simulink model "TRN_V3_2"  (R2022a)
settings: Solver=FixedStepAuto  StartTime=0.0  StopTime=300  FixedStep=0.04  RelTol=1e-3
PreLoadFcn:
  | load('BusStructureTRNsensor.mat');
  | addpath('C:/MAP');
InitFcn:
  | %load TRNDataBusPILS.mat
  | %addpath(genpath(cd))
  | 
  | %load('TPF_WHOLESIM_INPUT_SCENARIOS_AGCAS_N35_10E127_70.mat');
  | 
  | % Add DataBus Path
  | addpath(',,/');
  | addpath('../MAP/');
  | addpath('../MAP/MAP_DB');
  | addpath('../MAP/DVOF');
  | addpath(genpath(cd));
  | load('BusStructureTRN.mat');
undefined symbols (not defined in the file or in its folder): Altitude_INS, Latitude_INS, Longitude_INS, residual, Result_Prev, TimeTag_Prev, TRN, TRNlib
libraries: simulink_extras x21, sharedtransform x2
(part 3 of 4)

== system TRN_V3_2/TRN/ModeManagementCSU/TrackingCSU/TrackingCSU_20230430/TrackingCSU_Measurement/Measurement_GPSinvalid/residualValidCheck ==
  TRNDatapump : Inport
  Bus Selector7 : BusSelector  OutputSignals=residual
  Data Type Conversion2 : DataTypeConversion  OutDataTypeStr=boolean  SaturateOnIntegerOverflow=off  RndMeth=Floor
  Demux : Demux  Outputs=2
  Gain2 : Gain  Gain=3
  StdDev : MATLAB Function  TreatAsAtomicUnit=on
  Terminator : Terminator
  Unit Delay3 : UnitDelay  SampleTime=-1  HasFrameUpgradeWarning=on
  residualCheck : MATLAB Function  TreatAsAtomicUnit=on
  residualValid : Outport
  wires:
  Data Type Conversion2/1 -> residualValid/1
  residualCheck/1(residualValid) -> Data Type Conversion2/1
  StdDev/1(std) -> Gain2/1
  Gain2/1 -> residualCheck/2(sigma_3)
  residualCheck/2(count) -> Unit Delay3/1
  TRNDatapump/1 -> Bus Selector7/1
  Unit Delay3/1 -> residualCheck/3("count ")
  Bus Selector7/1 -> Demux/1  "<residual>"
  Demux/1 -> residualCheck/1(residual), StdDev/1(x)
  Demux/2 -> Terminator/1

== system TRN_V3_2/TRN/ModeManagementCSU/TrackingCSU/TrackingCSU_20230430/TrackingCSU_Measurement/Measurement_GPSvalid/residualValidCheck ==
  TRNDatapump : Inport
  Bus Selector7 : BusSelector  OutputSignals=residual
  Data Type Conversion2 : DataTypeConversion  OutDataTypeStr=boolean  SaturateOnIntegerOverflow=off  RndMeth=Floor
  Demux : Demux  Outputs=2
  Gain2 : Gain  Gain=3
  StdDev : MATLAB Function  TreatAsAtomicUnit=on
  Terminator : Terminator
  Unit Delay3 : UnitDelay  SampleTime=-1  HasFrameUpgradeWarning=on
  residualCheck : MATLAB Function  TreatAsAtomicUnit=on
  residualValid : Outport
  wires:
  Unit Delay3/1 -> residualCheck/3("count ")
  TRNDatapump/1 -> Bus Selector7/1
  residualCheck/2(count) -> Unit Delay3/1
  Gain2/1 -> residualCheck/2(sigma_3)
  StdDev/1(std) -> Gain2/1
  residualCheck/1(residualValid) -> Data Type Conversion2/1
  Data Type Conversion2/1 -> residualValid/1
  Bus Selector7/1 -> Demux/1  "<residual>"
  Demux/2 -> residualCheck/1(residual), StdDev/1(x)
  Demux/1 -> Terminator/1

== matlab function TRN_V3_2/TRN/ModeManagementCSU/TrackingCSU/TrackingCSU_20230430/TrackingCSU_ConvertInput1/GPSflagcheck ==
  data: FoM input; GPSflag output; GPSDataNotValid input; AccY input
function GPSflag  = GPScheck(FoM, GPSDataNotValid, AccY)

GPSflag = uint32(2);

if GPSDataNotValid == 0
%     if EstHorErr < 100 && EstVerErr < 25 && state == 5
        if FoM <= 4
            GPSflag = uint32(1);
            if FoM <= 2 && abs(AccY) < 2
                GPSflag = uint32(0);
            end
        end
%    end
else
    GPSflag = uint32(2);
end

== matlab function TRN_V3_2/TRN/ModeManagementCSU/TrackingCSU/TrackingCSU_20230430/TrackingCSU_Measurement/Measurement_GPSinvalid/MATLAB Function ==
  data: Rmat output
function Rmat = Rmatrix_GPSinvalid

% Original
% Rmat = diag((35/sqrt(25))^2);

% Monte-carlo simulation 972
% use min data
Rmat = diag((12.0679/sqrt(25))^2);

% Monte-carlo simulation 972
% use mean data
% Rmat = diag((9.9924/sqrt(25))^2);

== matlab function TRN_V3_2/TRN/ModeManagementCSU/TrackingCSU/TrackingCSU_20230430/TrackingCSU_EKFupdate1/EKFUpdate_GPSinvalid/EKFUpdate_GPSinvalid1 ==
  data: zmat_TRN input; xu output; P output; Fmatrix input; Hmat_TRN input; Gmatrix input; P input; Q input; Rmat_TRN input; dt input; residual output; latINSErrTRN output; lonINSErrTRN output; altINSErrTRN output; xu_prev input; TimeTag_Prev input; hUncertainty output; vUncertainty output
function [xu, P, residual, latINSErrTRN, lonINSErrTRN, altINSErrTRN, hUncertainty, vUncertainty] ...
    = EKFUpdate_GPSinvalid(zmat_TRN, Fmatrix, Hmat_TRN, Gmatrix, P, Q, Rmat_TRN, dt, xu_prev, TimeTag_Prev)

x = zeros(15,1);
I = eye(max(size(Fmatrix)));

A = I + (Fmatrix*dt);
Q = (A*Gmatrix * Q * Gmatrix'*A') .* dt;

%-------------------------------------%
% Predicts states & covariance matrix
%-------------------------------------%
xp = A * x;
Pp = (A * P * A') + Q;


K = (Pp * Hmat_TRN')/(Rmat_TRN + Hmat_TRN * Pp * Hmat_TRN');
xu = xp + K * (zmat_TRN - Hmat_TRN*xp);
residual = zmat_TRN;
P = (I - K*Hmat_TRN) * Pp * (I - K*Hmat_TRN)' + K*Rmat_TRN*K';

hUncertainty = sqrt(abs(P(7,7) + P(8,8))) * 6378000;    % unit m
vUncertainty = sqrt(abs(P(9,9)));                       % unit m

%---------------------------%
% Updates covariance matrix
%---------------------------%
% P = (I - K*H) * Pp * (I - K*H)' + K*R*K';

latINSErrTRN = xu(7);
lonINSErrTRN = xu(8);
altINSErrTRN = xu(9);

if (TimeTag_Prev(6) == 1)
    xu = xu_prev;
    latINSErrTRN = xu(7);
    lonINSErrTRN = xu(8);
    altINSErrTRN = xu(9);
end

== matlab function TRN_V3_2/TRN/ModeManagementCSU/TrackingCSU/TrackingCSU_20230430/TrackingCSU_Measurement/Measurement_GPSvalid/Rmat_GPS_v1 ==
  data: FoM input; Rmat output
% Original

function Rmat = Rmat_GPS(FoM)
Pcode = false;
if Pcode == true
    a = 6.4029;
    b = 6.7450;
    c = 8.8381;
    d = 0.8866;
    e = 1.1000;
    f = 3.3142;
elseif FoM == 1
    a = 6.4266;
    b = 6.7548;
    c = 17.6319;
    d = 0.8866;
    e = 1.1000;
    f = 3.3142;
elseif FoM == 2
    a = 6.5362;
    b = 6.8383;
    c = 34.2994;
    d = 0.8866;
    e = 1.1000;
    f = 3.3142;
elseif FoM == 3
    a = 6.7864;
    b = 7.0654;
    c = 55.6432;
    d = 0.8866;
    e = 1.1000;
    f = 3.3142;
elseif FoM == 4
    a = 7.1520;
    b = 7.4164;
    c = 77.1714;
    d = 0.8866;
    e = 1.1000;
    f = 3.3142;
else
    a = 8.6486;
    b = 8.8154;
    c = 135.9654;
    d = 0.8866;
    e = 1.1000;
    f = 3.3142;
end

Rmat = diag([ (a/sqrt(25))^2 (b/sqrt(25))^2 (c/sqrt(25))^2 (d/sqrt(25))^2 (e/sqrt(25))^2 (f/sqrt(25))^2 ]);

% Rmat = diag([ (6.6/sqrt(25))^2 (6.6/sqrt(25))^2 (1/sqrt(25))^2 (0.5/sqrt(25))^2 (0.5/sqrt(25))^2 (0.5/sqrt(25))^2 ]);

== matlab function TRN_V3_2/TRN/ModeManagementCSU/TrackingCSU/TrackingCSU_20230430/TrackingCSU_EKFupdate1/EKFUpdate_GPSinvalid/EKFUpdate_Predict_GPSinvalid ==
  data: I output; Zmat_GPSinvalid input; xp output; Pp output; Fmatrix input; Hmat_GPSinvalid input; Gmatrix input; P input; Q input; Rmat_GPSinvalid input; dt input; residual_GPSinvalid output; K output
function [I, xp, Pp, residual_GPSinvalid, K] ...
    = EKFUpdate_Predict_GPSinvalid(Zmat_GPSinvalid, Fmatrix, Hmat_GPSinvalid, Gmatrix, P, Q, Rmat_GPSinvalid, dt)

x = zeros(15,1);
I = eye(max(size(Fmatrix)));

A = I + (Fmatrix*dt);
Q = (A*Gmatrix * Q * Gmatrix'*A') .* dt;

%-------------------------------------%
% Predicts states & covariance matrix
%-------------------------------------%
xp = A * x;
Pp = (A * P * A') + Q;


K = (Pp * Hmat_GPSinvalid')/(Rmat_GPSinvalid + Hmat_GPSinvalid * Pp * Hmat_GPSinvalid');
residual_GPSinvalid = Zmat_GPSinvalid;

== matlab function TRN_V3_2/TRN/ModeManagementCSU/TrackingCSU/TrackingCSU_20230430/TrackingCSU_Measurement/Measurement_GPSvalid/Rmat_GPS_v2 ==
  data: FoM input; Rmat output
% Monte-carlo simulation 972
% use mean data

function Rmat = Rmat_GPS(FoM)
Pcode = false;
if Pcode == true
    a = 45.9175;
    b = 46.6241;
    c = 10.2589;
    d = 0.1085;
    e = 0.1108;
    f = 0.5579;
elseif FoM == 1
    a = 46.7399;
    b = 47.4166;
    c = 18.7833;
    d = 0.1085;
    e = 0.1108;
    f = 0.5579;
elseif FoM == 2
    a = 49.2325;
    b = 49.8506;
    c = 35.6076;
    d = 0.1085;
    e = 0.1108;
    f = 0.5579;
elseif FoM == 3
    a = 53.5206;
    b = 54.0688;
    c = 56.2876;
    d = 0.1085;
    e = 0.1108;
    f = 0.5579;
elseif FoM == 4
    a = 58.8912;
    b = 59.3679;
    c = 77.2285;
    d = 0.1085;
    e = 0.1108;
    f = 0.5579;
else
    a = 58.8912;
    b = 59.3679;
    c = 77.2285;
    d = 0.1085;
    e = 0.1108;
    f = 0.5579;
end

Rmat = diag([ (a/sqrt(25))^2 (b/sqrt(25))^2 (c/sqrt(25))^2 (d/sqrt(25))^2 (e/sqrt(25))^2 (f/sqrt(25))^2 ]);

== matlab function TRN_V3_2/TRN/ModeManagementCSU/ValidityCheck/ValidityCheck ==
  data: continuousValid input; TRNEstOfINSLatitudeErr output; TRNEstOfINSLongitudeErr output; TRNEstOfINSAltitudeErr output; AircraftPositionCorrectionValid output; latINSErrTRN input; lonINSErrTRN input; altINSErrTRN input; velFlag input
function [TRNEstOfINSLatitudeErr, TRNEstOfINSLongitudeErr, TRNEstOfINSAltitudeErr, AircraftPositionCorrectionValid] = ...
    ValidityCheck(continuousValid, latINSErrTRN, lonINSErrTRN, altINSErrTRN, velFlag)

if continuousValid == true || velFlag == true
    TRNEstOfINSLatitudeErr = latINSErrTRN * 180/pi;
    TRNEstOfINSLongitudeErr = lonINSErrTRN * 180/pi;
    TRNEstOfINSAltitudeErr = altINSErrTRN;
    AircraftPositionCorrectionValid = true;
else
    TRNEstOfINSLatitudeErr = 0.0;
    TRNEstOfINSLongitudeErr = 0.0;
    TRNEstOfINSAltitudeErr = 0.0;
    AircraftPositionCorrectionValid = false;
end
end

== matlab function TRN_V3_2/TRN/ModeManagementCSU/TrackingCSU/TrackingCSU_20230430/TrackingCSU_Measurement/Fupdate ==
  data: velN input; Fmatrix output; velE input; velD input; lat input; alt input; accN input; accE input; accD input; OM input; M input; N input; DCMbn input
% ---------------------------------------------------------------------- %
%                   F matrix update function
%
%   INPUT:
%       velN: North Velocity                                [m/s]
%       velE: East Velocity                                 [m/s]
%       velD: Down Velocity                                 [m/s]
%       lat: Latitude                                       [rad]
%       alt: Altitude                                       [m]
%       accN: North acceleration                            [m/ss]
%       accE: East acceleration                             [m/ss]
%       accD: Down acceleration                             [m/ss]
%       OM: Magnitude of the rotation rate of the Earth     [rad/s]
%       R0: Radius of Earth                                 [m]
%       DCMbn: Rotational matrix(body frame to navigation frame)
%
%   OUTPUT:
%       Fmatrix: System matrix of Kalman Filter
%
% ---------------------------------------------------------------------- %
function Fmatrix = Fupdate(velN, velE, velD, lat, alt, accN, accE, accD, OM, M, N, DCMbn)
    
        Z  = zeros(3);
    
        e11 = 0;
        e12 = -((OM * sin(lat)) + (velE/(N+alt) * tan(lat)));
        e13 = velN/(M+alt);
        e21 = ((OM * sin(lat)) + (velE/(N+alt) * tan(lat)));
        e22 = 0;
        e23 = ((OM * cos(lat)) + (velE/(N+alt)));
        e31 = -velN/(M+alt);
        e32 = -(OM * cos(lat)) - (velE/(N+alt));
        e33 = 0;
        Fee = [e11 e12 e13; e21 e22 e23; e31 e32 e33;];
    
        e11 = 0;
        e12 = 1/((N+alt));
        e13 = 0;
        e21 = -1/((M+alt));
        e22 = 0 ;
        e23 = 0 ;
        e31 = 0 ;
        e32 = -tan(lat)/(N+alt) ;
        e33 = 0 ;
        Fev = [e11 e12 e13; e21 e22 e23; e31 e32 e33;];
    
        e11 = -OM * sin(lat);
        e12 = 0;
        e13 = -velE/(((N+alt))^2);
        e21 = 0 ;
        e22 = 0 ;
        e23 = velN/(((M+alt))^2);
        e31 =  -(OM*cos(lat)) - (velE/(((N+alt))*(cos(lat))^2));
        e32 = 0 ;
        e33 = (velE * tan(lat)) / ((N+alt)^2) ;
        Fep = [e11 e12 e13; e21 e22 e23; e31 e32 e33;];
    
        e11 = 0 ;
        e12 = -accD ;
        e13 = accE ;
        e21 = accD ;
        e22 = 0 ;
        e23 = -accN ;
        e31 = -accE ;
        e32 = accN ;
        e33 = 0 ;
        Fve = [e11 e12 e13; e21 e22 e23; e31 e32 e33;];
    
        e11 = velD/((M+alt));
        e12 = -2*((OM * sin(lat)) + ((velE/((N+alt))) * tan (lat))) ;
        e13 = velN/(M+alt) ;
        e21 = (2*OM * sin(lat)) + ( (velE/((N+alt))) * tan(lat) );
        e22 = (1/((N+alt))) * ((velN * tan(lat)) + velD) ;
        e23 = 2*OM * cos(lat) + (velE/((N+alt)));
        e31 = (-2*velN)/((M+alt));
        e32 = -2*(OM * cos(lat) +  (velE/((N+alt)))) ;
        e33 = 0;
        Fvv = [e11 e12 e13; e21 e22 e23; e31 e32 e33;];
    
        e11 = -velE*( (2*OM * cos(lat)) + (velE/(((N+alt))*(cos(lat))^2)));
        e12 = 0 ;
        e13 = (((velE^2)*tan(lat))/((N+alt)^2)) - ((velN*velD)/((M+alt)^2)) ;
        e21 = 2*OM *((velN*cos(lat)) - (velD*sin(lat))) + ((velN*velE) / (((N+alt))*(cos(lat))^2)) ;
        e22 = 0 ;
        e23 = ((-velE*velD)/((N+alt)^2))-((velN*velE*tan(lat))/((N+alt)^2));
        e31 = 2 * OM * velE * sin(lat);
        e32 = 0;
        e33 =  (((velE^2)/((N+alt)^2)) + ((velN^2)/((M+alt)^2)));
        Fvp = [e11 e12 e13; e21 e22 e23; e31 e32 e33;];
    
        Fpe = zeros(3);
    
        e11 = 1/((M+alt));
        e12 = 0;
        e13 = 0;
        e21 = 0;
        e22 = 1/(((N+alt))*cos(lat));
        e23 = 0;
        e31 = 0;
        e32 = 0;
        e33 = -1;
        Fpv = [e11 e12 e13; e21 e22 e23; e31 e32 e33;];
    
        e11 = 0;
        e12 = 0;
        e13 = -velN/(((M+alt))^2);
        e21 = (velE*tan(lat))/(((N+alt))*cos(lat));
        e22 = 0;
        e23 = -velE/((((N+alt))^2)*cos(lat));
        e31 = 0;
        e32 = 0;
        e33 = 0;
        Fpp = [e11 e12 e13; e21 e22 e23; e31 e32 e33;];
    
    
        %     Fvv = zeros(3);
        %     Fvp = zeros(3);
        %     Fpp = zeros(3);
    
        Fmatrix =  [Fee    Fev    Fep      DCMbn          Z      ;
                    Fve    Fvv    Fvp        Z           DCMbn   ;
                    Fpe    Fpv    Fpp        Z            Z      ;
                    Z      Z      Z          Z            Z      ;
                    Z      Z      Z          Z            Z      ;];


end

== matlab function TRN_V3_2/TRN/ModeManagementCSU/TrackingCSU/TrackingCSU_20230430/TrackingCSU_Measurement/Gupdate ==
  data: DCMbn input; Gmatrix output
% ---------------------------------------------------------------------- %
%                   G matrix update function
%
%   INPUT:
%       DCMbn: Rotational matrix(body frame to navigation frame)
%
%   OUTPUT:
%       Gmatrix: Input matrix of Kalman Filter
%
% ---------------------------------------------------------------------- %
function Gmatrix = Gupdate(DCMbn)

Z  = zeros(3);

Gmatrix =  [ -DCMbn     Z;
                Z      DCMbn;
                Z       Z;
                Z       Z;
                Z       Z;];      

end

== matlab function TRN_V3_2/TRN/ModeManagementCSU/TrackingCSU/TrackingCSU_20230430/TrackingCSU_Measurement/Measurement_GPSinvalid/MesurementUpdate_GPSinvalid ==
  data: Hmat_GPSinvalid output; lat input; lon input; alt input; RALTAltitude input; Zmat_GPSinvalid output; resolution input
% function [Hmatrix, z, hDEM] = MeasurementUpdate(resolution, lat, lon, alt, RALT)
function [Hmat_GPSinvalid, Zmat_GPSinvalid] = MeasurementUpdate(lat, lon, alt, RALTAltitude, resolution)
    P_low = 0.0;
    P_high = 0.0;    
    P_left = 0.0;    
    P_right = 0.0;
    hDEM = double(0.0);         
    resultDTED = uint32(1);

    lat = rad2deg(lat);
    lon = rad2deg(lon);

    resultDTED = coder.ceval('UpdateCache', lat, lon);
    
    P_low    =   coder.ceval('MAPGetTerrainHeight', lat - resolution, lon);
    P_high   =   coder.ceval('MAPGetTerrainHeight', lat + resolution, lon);
    P_left   =   coder.ceval('MAPGetTerrainHeight', lat, lon - resolution);
    P_right  =   coder.ceval('MAPGetTerrainHeight', lat, lon + resolution);
    
    hdot_lat    =   (P_high - P_low) / (resolution);
    hdot_lon    =   (P_right - P_left) / (resolution);
    
    % H matrix
    Hmat_GPSinvalid = [ zeros(1,6) -hdot_lat   -hdot_lon    1  zeros(1,6) ]; 
    
    hDEM = coder.ceval('MAPGetTerrainHeight', lat, lon);
    
    Zmat_GPSinvalid = (alt - hDEM) - RALTAltitude;

end

== matlab function TRN_V3_2/TRN/ModeManagementCSU/TrackingCSU/TrackingCSU_20230430/TrackingCSU_Measurement/Measurement_GPSinvalid/MesurementValid_GPSinvalid ==
  data: updateValid input; roll input; pitch input; zmat_out output; zmat_in input; RALTTimeTag input; RALTTimeTag_temp input; RLATvalid input
function zmat_out  = MesurementValid(updateValid, roll, pitch, zmat_in, RALTTimeTag, RALTTimeTag_temp, RLATvalid)

zmat_out = 0;

if (updateValid == true && abs(roll) < deg2rad(15) && abs(pitch) < deg2rad(15) && RLATvalid == true && (abs(RALTTimeTag - RALTTimeTag_temp)) ~= 0)
% if (residualValid == true && abs(roll) < deg2rad(15) && abs(pitch) < deg2rad(15) && (abs(RALTTimeTag - RALTTimeTag_temp)) > 0.000000001)
% if (RALTValid == true && abs(roll) < deg2rad(15) && abs(pitch) < deg2rad(15))
    zmat_out = zmat_in;


else
    zmat_out = 0;

end

end

== matlab function TRN_V3_2/TRN/ModeManagementCSU/TrackingCSU/TrackingCSU_20230430/TrackingCSU_Measurement/Measurement_GPSinvalid/residualValidCheck/StdDev ==
  data: x input; std output
function std = StdDev(x)

persistent sumX sumX2 cnt
if (isempty(sumX))
    sumX = 0;
end
if (isempty(sumX2))
    sumX2 = 0;
end
if (isempty(cnt))
    cnt = 0;
end

cnt = cnt + 1;
sumX = sumX + x;
sumX2 = sumX2 + x^2;

var = sumX2/cnt - (sumX/cnt)^2;
std = sqrt(abs(var));
end

== matlab function TRN_V3_2/TRN/ModeManagementCSU/TrackingCSU/TrackingCSU_20230430/TrackingCSU_Measurement/Measurement_GPSinvalid/residualValidCheck/residualCheck ==
  data: residual input; sigma_3 input; residualValid output; count output; count input
function [residualValid, count] = residualCheck(residual, sigma_3, count)

if abs(residual) > sigma_3
    count = count + 1;
else
    count = 0;
end

if count > 7
    residualValid = boolean(false);
else
    residualValid = boolean(true);
end

== matlab function TRN_V3_2/TRN/ModeManagementCSU/TrackingCSU/TrackingCSU_20230430/TrackingCSU_Measurement/Measurement_GPSvalid/Earth_radius ==
  data: M output; N output; psi output; Latitude_INS input
function [M, N, psi] = Earth_radius(Latitude_INS)

    a   = 6378137;          % Earth's equatorial radius
    b   = 6356752.314245;   % Earth's polar radius
    psi = Latitude_INS;     % psi(latitude_INS)
    M   = ((a*b)^2) / ( ( (a*cos(psi))^2 + (b*sin(psi))^2 )^(3/2) );    % radius  of  curvature  in  meridian
    N   = (a^2) / ( ( (a*cos(psi))^2 + (b*sin(psi))^2 )^(1/2) );        % radius  of  curvature  in  prime  vertical

end

== matlab function TRN_V3_2/TRN/ModeManagementCSU/TrackingCSU/TrackingCSU_20230430/TrackingCSU_Measurement/Measurement_GPSvalid/MesurementUpdate_GPSvalid ==
  data: Lat_GPS input; Hmat_GPSvalid output; Lon_GPS input; z_GPSvalid output; Alt_GPS input; velN_GPS input; velE_GPS input; velD_GPS input; Lat_INS input; Lon_INS input; Alt_INS input; velN_INS input; velE_INS input; velD_INS input; M input; N input; psi input
function [Hmat_GPSvalid, z_GPSvalid] = MeasurementUpdate(Lat_GPS, Lon_GPS, Alt_GPS, velN_GPS, velE_GPS, velD_GPS, ...
                                          Lat_INS, Lon_INS, Alt_INS, velN_INS, velE_INS, velD_INS, ...
                                          M, N, psi)
    Z   = zeros(3);
    I   = eye(3);
    H   = [(M+Alt_INS)        0             0;
        0     (N+Alt_INS)*cos(psi)     0;
        0            0             1];

    % H matrix
    Hmat_GPSvalid = [Z Z H Z Z
                   Z I Z Z Z];


    z_GPSvalid = [(M+Alt_INS)*(Lat_INS-Lat_GPS);
        (N+Alt_INS)*cos(psi)*(Lon_INS-Lon_GPS);
        Alt_INS - Alt_GPS;
        velN_INS - velN_GPS;
        velE_INS - velE_GPS;
        velD_INS - velD_GPS];

end

== matlab function TRN_V3_2/TRN/ModeManagementCSU/TrackingCSU/TrackingCSU_20230430/TrackingCSU_Measurement/Measurement_GPSvalid/MesurementValid_GPSvalid ==
  data: zmat_in_GPSvalid input; roll input; pitch input; zmat_GPSvalid output; GPStimeValid input; GPStimeValid_temp input; GPS_flag input; residualValid input
function zmat_GPSvalid = MesurementValid(zmat_in_GPSvalid,  roll, pitch, GPStimeValid, GPStimeValid_temp, GPS_flag, residualValid)

zmat_GPSvalid = zeros(6,1);

if (residualValid == true && abs(roll) < deg2rad(15) && abs(pitch) < deg2rad(15) && (abs(GPStimeValid - GPStimeValid_temp)) ~= 0)
    %     if (residualValid == true) && (abs(GPStimeValid - GPStimeValid_temp) > 0.000000001)

    if GPS_flag == 0
        zmat_GPSvalid = zmat_in_GPSvalid;

    elseif GPS_flag == 1

        for i = 1:6
            zmat_GPSvalid(i) = zmat_in_GPSvalid(i);

            if i > 3
                zmat_GPSvalid(i) = 0;
            end
        end

    else
        zmat_GPSvalid = zeros(6,1);
    end

else
    zmat_GPSvalid = zeros(6,1);

end

end

== matlab function TRN_V3_2/TRN/ModeManagementCSU/TrackingCSU/TrackingCSU_20230430/TrackingCSU_Measurement/Measurement_GPSvalid/residualValidCheck/StdDev ==
  data: x input; std output
function std = StdDev(x)

persistent sumX sumX2 cnt
if (isempty(sumX))
    sumX = 0;
end
if (isempty(sumX2))
    sumX2 = 0;
end
if (isempty(cnt))
    cnt = 0;
end

cnt = cnt + 1;
sumX = sumX + x;
sumX2 = sumX2 + x^2;

var = sumX2/cnt - (sumX/cnt)^2;
std = sqrt(abs(var));
end

== matlab function TRN_V3_2/TRN/ModeManagementCSU/TrackingCSU/TrackingCSU_20230430/TrackingCSU_Measurement/Measurement_GPSvalid/residualValidCheck/residualCheck ==
  data: residual input; sigma_3 input; residualValid output; count output; count input
function [residualValid, count] = residualCheck(residual, sigma_3, count)

if abs(residual) > sigma_3
    count = count + 1;
else
    count = 0;
end

if count > 7
    residualValid = boolean(false);
else
    residualValid = boolean(true);
end

== matlab function TRN_V3_2/TRN/ModeManagementCSU/TrackingCSU/TrackingCSU_20230430/TrackingCSU_Measurement/Measurement_GPSvalid/Rmat_GPS_v3 ==
  data: FoM input; Rmat output
% Monte-carlo simulation 972
% use min data

function Rmat = Rmat_GPS(FoM)
Pcode = false;
if Pcode == true
    a = 4.0773;
    b = 3.4166;
    c = 8.0620;
    d = 0.0913;
    e = 0.0866;
    f = 0.4882;
elseif FoM == 1
    a = 7.6366;
    b = 7.1937;
    c = 16.1792;
    d = 0.0913;
    e = 0.0866;
    f = 0.4882;
elseif FoM == 2
    a = 14.4437;
    b = 14.1249;
    c = 31.3340;
    d = 0.0913;
    e = 0.0866;
    f = 0.4882;
elseif FoM == 3
    a = 23.1033;
    b = 22.5088;
    c = 49.8294;
    d = 0.0913;
    e = 0.0866;
    f = 0.4882;
elseif FoM == 4
    a = 31.8984;
    b = 30.9599;
    c = 68.6016;
    d = 0.0913;
    e = 0.0866;
    f = 0.4882;
else
    a = 31.8984;
    b = 30.9599;
    c = 68.6016;
    d = 0.0913;
    e = 0.0866;
    f = 0.4882;
end

Rmat = diag([ (a/sqrt(25))^2 (b/sqrt(25))^2 (c/sqrt(25))^2 (d/sqrt(25))^2 (e/sqrt(25))^2 (f/sqrt(25))^2 ]);

== matlab function TRN_V3_2/TRN/ModeManagementCSU/Ver_FlightPath_Angle/FlightPath_Angle ==
  data: vNED input; TRN_Ver_FlightPath_Angle output
function TRN_Ver_FlightPath_Angle  = FlightPath_Angle(vNED)

vN = vNED(1);
vE = vNED(2);
vD = vNED(3);

TRN_Ver_FlightPath_Angle = atan(-vD/sqrt(vN^2+vE^2));

== matlab function TRN_V3_2/TRN/TRNCorrCheck ==
  data: latINS input; TRNEstOfLatErr output; lonINS input; altINS input; TRNEstOfLonErr output; TRNEstOfaltErr output; roll input; pitch input; GPSDataNotvalid input; NotCorrFlag input; NotCorrFlag output
function [TRNEstOfLatErr, TRNEstOfLonErr, TRNEstOfaltErr,NotCorrFlag] = TRNCorrCheck(latINS, lonINS, altINS, roll, pitch, GPSDataNotvalid, NotCorrFlag)

% if GPSDataNotvalid == true
%     if abs(roll) > 15 || abs(pitch) > 15
%         TRNEstOfLatErr_temp = latINS;
%         TRNEstOfLonErr_temp = lonINS;
%         TRNEstOfaltErr_temp = altINS;
%         TRNEstOfLatErr = TRNEstOfLatErr_temp;
%         TRNEstOfLonErr = TRNEstOfLonErr_temp;
%         TRNEstOfaltErr = TRNEstOfaltErr_temp;
%         NotCorrFlag = 1;
%     else
%         TRNEstOfLatErr = latINS;
%         TRNEstOfLonErr = lonINS;
%         TRNEstOfaltErr = altINS;
%         TRNEstOfLatErr_temp = 0;
%         TRNEstOfLonErr_temp = 0;
%         TRNEstOfaltErr_temp = 0;
%         NotCorrFlag = 0;
%     end
%     
%     if NotCorrFlag == 1
%         TRNEstOfLatErr = TRNEstOfLatErr_temp;
%         TRNEstOfLonErr = TRNEstOfLonErr_temp;
%         TRNEstOfaltErr = TRNEstOfaltErr_temp;
%     end
% else
    TRNEstOfLatErr = latINS;
    TRNEstOfLonErr = lonINS;
    TRNEstOfaltErr = altINS;
    NotCorrFlag = 0;
% end

== matlab function TRN_V3_2/TRN/TRNEventInjector1 ==
  data: inBus input Bus: TRNOutput; outBus output Bus: TRNOutput
function outBus = TRNEventInjector(inBus)
persistent time dt
if isempty(time)
    time = 0.0;
end
if isempty(dt)
    dt = 0.04;
end

Activated = false;

outBus = inBus;

if Activated
    if (30 <= time) && (time < 31)
        outBus.TRN_valid = false;
    elseif (40 <= time) && (time < 41)
        outBus.AircraftPositionCorrectionValid = false;
    elseif (50 <= time) && (time < 51)
        outBus.AircraftOffTerrainMap = true;
    elseif (40 <= time) && (time < 41)
        outBus.NavigationMode = true;
    elseif (70 <= time) && (time <73)
        outBus.TRN_VelocityX = 30;
        outBus.TRN_VelocityY = 0;
        outBus.TRN_VelocityZ = 0;
    end
end

time = time + dt;

== matlab function TRN_V3_2/TRN/ModeManagementCSU/TrackingCSU/TrackingCSU_20230430/TrackingCSU_EKFupdate1/EKFUpdate_GPSinvalid/EKFUpdate_Update_GPSinvalid ==
  data: I input; xu_GPSinvalid output; P_GPSinvalid output; xp input; Pp input; latINSErrTRN_GPSinvalid output; lonINSErrTRN_GPSinvalid output; altINSErrTRN_GPSinvalid output; K input; Zmat_GPSinvalid input; Hmat_GPSinvalid input; Rmat_GPSinvalid input; xu_prev_GPSinvalid input; TimeTag_Prev input; hUncertainty_GPSinvalid output; vUncertainty_GPSinvalid output
function [xu_GPSinvalid, P_GPSinvalid, latINSErrTRN_GPSinvalid, lonINSErrTRN_GPSinvalid, altINSErrTRN_GPSinvalid, hUncertainty_GPSinvalid, vUncertainty_GPSinvalid] ...
    = EKFUpdate_Update_GPSinvalid(I, xp, Pp, K, Zmat_GPSinvalid, Hmat_GPSinvalid, Rmat_GPSinvalid, xu_prev_GPSinvalid, TimeTag_Prev)

xu_GPSinvalid = xp + K * (Zmat_GPSinvalid - Hmat_GPSinvalid*xp);
P_GPSinvalid = (I - K*Hmat_GPSinvalid) * Pp * (I - K*Hmat_GPSinvalid)' + K*Rmat_GPSinvalid*K';

hUncertainty_GPSinvalid = sqrt(abs(P_GPSinvalid(7,7) + P_GPSinvalid(8,8))) * 6378000;    % unit m
vUncertainty_GPSinvalid = sqrt(abs(P_GPSinvalid(9,9)));                       % unit m

latINSErrTRN_GPSinvalid = xu_GPSinvalid(7);
lonINSErrTRN_GPSinvalid = xu_GPSinvalid(8);
altINSErrTRN_GPSinvalid = xu_GPSinvalid(9);

if (TimeTag_Prev(6) == 1)
    xu_GPSinvalid = xu_prev_GPSinvalid;
    latINSErrTRN_GPSinvalid = xu_GPSinvalid(7);
    lonINSErrTRN_GPSinvalid = xu_GPSinvalid(8);
    altINSErrTRN_GPSinvalid = xu_GPSinvalid(9);
end

== matlab function TRN_V3_2/TRN/ModeManagementCSU/TrackingCSU/TrackingCSU_20230430/TrackingCSU_EKFupdate1/EKFUpdate_GPSvalid/EKFUpdate_Kgain_GPSvalid ==
  data: Hmat_GPSvalid input; Rmat_GPSvalid input; Pp input; K output
function K = EKFUpdate_Kgain_GPSvalid( Hmat_GPSvalid, Rmat_GPSvalid, Pp)


K = (Pp * Hmat_GPSvalid')/(Rmat_GPSvalid + Hmat_GPSvalid * Pp * Hmat_GPSvalid');




end

== matlab function TRN_V3_2/TRN/ModeManagementCSU/TrackingCSU/TrackingCSU_20230430/TrackingCSU_EKFupdate1/EKFUpdate_GPSvalid/EKFUpdate_Predict_GPSvalid ==
  data: I output; xp output; Pp output; Fmatrix input; Gmatrix input; P input; Q input; dt input; Zmat_GPSvalid input; residual_GPSvalid output
function [I, xp, Pp, residual_GPSvalid] ...
    = EKFUpdate_Predict_GPSvalid(Fmatrix, Gmatrix, P, Q, dt, Zmat_GPSvalid)

x = zeros(15,1);
I = eye(max(size(Fmatrix)));

A = I + (Fmatrix*dt);
Q = (A*Gmatrix * Q * Gmatrix'*A') .* dt;

%-------------------------------------%
% Predicts states & covariance matrix
%-------------------------------------%
xp = A * x;
Pp = (A * P * A') + Q;
residual_GPSvalid = Zmat_GPSvalid(3);

end

== matlab function TRN_V3_2/TRN/ModeManagementCSU/TrackingCSU/TrackingCSU_20230430/TrackingCSU_EKFupdate1/EKFUpdate_GPSvalid/EKFUpdate_Update_GPSvalid ==
  data: I input; xu_GPSvalid output; P_GPSvalid output; xp input; Pp input; latINSErrTRN_GPSvalid output; lonINSErrTRN_GPSvalid output; altINSErrTRN_GPSvalid output; K input; Zmat_GPSvalid input; Hmat_GPSvalid input; Rmat_GPSvalid input; xu_prev_GPSvalid input; TimeTag_Prev input; hUncertainty_GPSvalid output; vUncertainty_GPSvalid output; GPSHorUncert input; GPSVerUncert input
function [xu_GPSvalid, P_GPSvalid, latINSErrTRN_GPSvalid, lonINSErrTRN_GPSvalid, altINSErrTRN_GPSvalid, hUncertainty_GPSvalid, vUncertainty_GPSvalid] ...
    = EKFUpdate_Update_GPSvalid(I, xp, Pp, K, Zmat_GPSvalid, Hmat_GPSvalid, Rmat_GPSvalid, xu_prev_GPSvalid, TimeTag_Prev, GPSHorUncert, GPSVerUncert)

xu_GPSvalid = xp + K * (Zmat_GPSvalid - Hmat_GPSvalid*xp);
P_GPSvalid = (I - K*Hmat_GPSvalid) * Pp * (I - K*Hmat_GPSvalid)' + K*Rmat_GPSvalid*K';

hUncertainty_GPSvalid = double(GPSHorUncert);     % unit m
vUncertainty_GPSvalid = double(GPSVerUncert);     % unit m


%---------------------------%
% Updates covariance matrix
%---------------------------%
% P = (I - K*H) * Pp * (I - K*H)' + K*R*K';

latINSErrTRN_GPSvalid = xu_GPSvalid(7);
lonINSErrTRN_GPSvalid = xu_GPSvalid(8);
altINSErrTRN_GPSvalid = xu_GPSvalid(9);
if (TimeTag_Prev(4) == 1)
    xu_GPSvalid = xu_prev_GPSvalid;
    latINSErrTRN_GPSvalid = xu_GPSvalid(7);
    lonINSErrTRN_GPSvalid = xu_GPSvalid(8);
    altINSErrTRN_GPSvalid = xu_GPSvalid(9);
end
%--------------------------------------------------------%

== matlab function TRN_V3_2/TRN/TRN_visualization/MATLAB Function ==
  data: TRN_valid input; TRNOperatingEnv_Flag output; roll input; pitch input; INSDataNotvalid input
function TRNOperatingEnv_Flag  = TRNCorrCheck(TRN_valid, roll, pitch, INSDataNotvalid)

if (TRN_valid == true) && (roll < 15) && (pitch < 15) && (INSDataNotvalid == true)
    TRNOperatingEnv_Flag = boolean(true);
else
    TRNOperatingEnv_Flag = boolean(false);
end


end

== matlab function TRN_V3_2/TRN/ModeManagementCSU/TrackingCSU/TrackingCSU_20230430/TrackingCSU_EKFupdate1/GPSWeight ==
  data: P_code input; C_code input; GPSFoM input; GPSWeight output
function GPSWeight = GPSWeight(P_code, C_code, GPSFoM)

if P_code == 1

    GPSWeight = [0.9899    0.9880    0.4535    0.9888];      % weight : lat, lon, alt, lat/lon squre root sum

elseif P_code == 0 && C_code == 1

    if GPSFoM == 1

        GPSWeight = [ 0.9899    0.9880    0.4535    0.9888];

    elseif  GPSFoM == 2

        GPSWeight = [ 0.9897    0.9879    0.3262    0.9887];

    elseif  GPSFoM == 3

        GPSWeight = [0.9894    0.9876    0.2470    0.9884];

    elseif  GPSFoM == 4

        GPSWeight = [0.9890    0.9872    0.2020    0.9880];

    else

        GPSWeight = [0.0 0.0 0.0 0.0];
    
    end

else

    GPSWeight = [0.0 0.0 0.0 0.0];

end

end

== matlab function TRN_V3_2/TRN/ModeManagementCSU/TrackingCSU/TrackingCSU_20230430/TrackingCSU_EKFupdate1/MATLAB Function2 ==
  data: P_GPSinvalid input; Pmat_GPSvalid output; Pmat_GPSinvalid output; P_GPSvalid input; Weight_GPSvalid output; Weight_GPSinvalid output
function [Pmat_GPSvalid, Pmat_GPSinvalid, Weight_GPSvalid, Weight_GPSinvalid] = fcn(P_GPSinvalid, P_GPSvalid)

Pmat_GPSvalid = zeros(1,3);
Pmat_GPSinvalid = zeros(1,3);
Weight_GPSvalid = zeros(1,3);
Weight_GPSinvalid = zeros(1,3);

for i = 7:8

    Pmat_GPSvalid(1,i-6)   = sqrt(P_GPSvalid(i,i)) * 6378000;
    Pmat_GPSinvalid(1,i-6) = sqrt(P_GPSinvalid(i,i)) * 6378000;

end

Pmat_GPSvalid(1,3)   = sqrt(P_GPSvalid(9,9));
Pmat_GPSinvalid(1,3) = sqrt(P_GPSinvalid(9,9));

for j = 1:3
    Weight_GPSvalid(j)   = Pmat_GPSinvalid(1,j) / (Pmat_GPSvalid(1,j) + Pmat_GPSinvalid(1,j));  % Pmat이 클수록 못믿음
    Weight_GPSinvalid(j) = 1 - Weight_GPSvalid(j);
end

== matlab function TRN_V3_2/TRN/ModeManagementCSU/TrackingCSU/TrackingCSU_20230430/TrackingCSU_EKFupdate1/weightCheck ==
  data: GPSWeight input; GPSflag input; weight output; GPSDataNotValid input
function weight = weightCheck(GPSWeight, GPSflag, GPSDataNotValid)

persistent GPSvalid2invalidCnt Weight_temp
if(isempty(GPSvalid2invalidCnt))
    GPSvalid2invalidCnt = 0.0;
end
if(isempty(Weight_temp))
    Weight_temp = [0.0 0.0 0.0 0.0];
end

if GPSflag > 1 || GPSDataNotValid == true           % GPS invalid

    if 30.0 <= GPSvalid2invalidCnt
       
        GPSvalid2invalidCnt = 30.0;

    end

    weight = Weight_temp .* (1 - GPSvalid2invalidCnt/30);
    GPSvalid2invalidCnt = GPSvalid2invalidCnt + 0.04;

else                                                % GPS valid     // GPS invalid > valid 시, 30초간 서서히 weight가 커지도록 구현 필요
    
    Weight_temp = GPSWeight;
    weight = GPSWeight;

    GPSvalid2invalidCnt = 0.0;
    
end

end

== matlab function TRN_V3_2/TRN/ModeManagementCSU/TrackingCSU/TrackingCSU_20230430/TrackingCSU_EKFupdate1/weighted sum ==
  data: GPSinvalid_errorMat input; weight input; GPSvalid_errorMat input; latINSErrTRN output; lonINSErrTRN output; altINSErrTRN output; hUncertainty output; vUncertainty output
function [latINSErrTRN, lonINSErrTRN, altINSErrTRN, hUncertainty, vUncertainty] = ...
          weightedSum(GPSinvalid_errorMat, weight, GPSvalid_errorMat)

%   GPSvalid_errorMat = [latINSErrTRN_GPSvalid,   lonINSErrTRN_GPSvalid,   altINSErrTRN_GPSvalid,   hUncertainty_GPSvalid,   vUncertainty_GPSvalid];
%   GPSinvalid_errorMat = [latINSErrTRN_GPSinvalid, lonINSErrTRN_GPSinvalid, altINSErrTRN_GPSinvalid, hUncertainty_GPSinvalid, vUncertainty_GPSinvalid];
%   weight = [lat lon alt (lat+lon squre root sum) alt]

latINSErrTRN = GPSvalid_errorMat(1) * weight(1) + GPSinvalid_errorMat(1) * ( 1 - weight(1) );

lonINSErrTRN = GPSvalid_errorMat(2) * weight(2) + GPSinvalid_errorMat(2) * ( 1 - weight(2) );

altINSErrTRN = GPSvalid_errorMat(3) * weight(3) + GPSinvalid_errorMat(3) * ( 1 - weight(3) );

hUncertainty = GPSvalid_errorMat(4) * weight(4) + GPSinvalid_errorMat(4) * ( 1 - weight(4) );

vUncertainty = GPSvalid_errorMat(5) * weight(3) + GPSinvalid_errorMat(5) * ( 1 - weight(3) );

end

== matlab function TRN_V3_2/TRN/ModeManagementCSU/AcquisitionCSU/AcquisitionCSU/CollectProfile ==
  data: profileCnt input; hDEM output; batchProfile output; batchProfile input; gridSize input; resolution input; gridRes input
function [hDEM,batchProfile]  = CollectProfile(profileCnt, batchProfile, gridSize, resolution, gridRes)

latTemp     = 0;
lonTemp     = 0;
hDEM        = 0;


for i = -gridSize : gridSize
    for j = -gridSize : gridSize
        
        latTemp = batchProfile(((profileCnt-1)*(3+(gridSize+gridSize+1)*(gridSize+gridSize+1))) + 2) + i*gridRes*resolution;
        lonTemp = batchProfile(((profileCnt-1)*(3+(gridSize+gridSize+1)*(gridSize+gridSize+1))) + 3) + j*gridRes*resolution;
        hDEM    = coder.ceval('MAPGetTerrainHeight', latTemp*180/pi, lonTemp*180/pi);

        batchProfile(((profileCnt-1)*(3+(gridSize+gridSize+1)*(gridSize+gridSize+1))) + 3 + ((i + gridSize) * (gridSize+gridSize+1)) + (j + gridSize + 1)) = abs(batchProfile(((profileCnt-1)*(3+(gridSize+gridSize+1)*(gridSize+gridSize+1))) + 1) - hDEM );   
    end
end



end

== matlab function TRN_V3_2/TRN/ModeManagementCSU/AcquisitionCSU/AcquisitionCSU/CorrelationAnalysis ==
  data: batchProfile input; profileCnt input; posUpdate output; MAD output; gridSize input; residual output; resolution input; gridRes input
function [posUpdate, MAD, residual] = CorrelationAnalysis(batchProfile, profileCnt, gridSize, resolution, gridRes)

MAD         = single(0);
bestIdx     = [-999 -999];
posUpdate   = zeros(2,1);
MADTemp     = 9999*ones(1,8000);
sum         = 0;

for i = 1 : (gridSize+gridSize+1) * (gridSize+gridSize+1)
    sum = 0;
    for j = 1 : profileCnt
        sum = sum + batchProfile(((j-1)*(3+(gridSize+gridSize+1)*(gridSize+gridSize+1))) + (i+3));
    end
    
    MADTemp(1,i) = sum/single(profileCnt);
    
end

[minMAD, minIdx] = min(MADTemp);
MAD = single(minMAD);

bestIdx(1) = floor(minIdx/(gridSize+gridSize+1));
bestIdx(2) = minIdx - (bestIdx(1) * (gridSize+gridSize+1));

if (IsNear(bestIdx(2), 0))
    bestIdx(1) = bestIdx(1) - 1;
    bestIdx(2) = (gridSize+gridSize);
end
%
bestIdx(1) = bestIdx(1) - gridSize;
bestIdx(2) = bestIdx(2) - gridSize - 1;
posUpdate(1) = bestIdx(1)*gridRes*resolution;
posUpdate(2) = bestIdx(2)*gridRes*resolution;

residual = double(MAD);

end


function tf=IsNear(a,b,tol)
%ISNEAR True Where Nearly Equal.
% ISNEAR(A,B) returns a logical array the same size as A and B that is True
% where A and B are almost equal to each other and False where they are not.
% A and B must be the same size or one can be a scalar.
% ISNEAR(A,B,TOL) uses the tolerance TOL to determine nearness. In this
% case, TOL can be a scalar or an array the same size as A and B.
%
% When TOL is not provided, TOL = SQRT(eps).
%
% Use this function instead of A==B when A and B contain noninteger values.
% D.C. Hanselman, University of Maine, Orono, ME 04469
% Mastering MATLAB 7
% 2005-03-09
%--------------------------------------------------------------------------
if nargin==2
%    tol=sqrt(eps);       % original version
	tol=sqrt(eps(max(abs(a),abs(b))));     %  my version. sqrt seems like 'overdamping'
end
% when in need of optimization, drop the error checks
if ~isnumeric(a) || isempty(a) || ~isnumeric(b) || isempty(b) ||...
   ~isnumeric(tol) || isempty(tol)
   error('Inputs Must be Numeric.')
end
if any(size(a)~=size(b)) && numel(a)>1 && numel(b)>1
   error('A and B Must be the Same Size or Either can be a Scalar.')
end
% main line
tf=abs((a-b))<=abs(tol);
end

== matlab function TRN_V3_2/TRN/ModeManagementCSU/AcquisitionCSU/AcquisitionCSU/MAPValid ==
  data: In_MAPValid input; MAPValid output
function MAPValid = MAPValid(In_MAPValid)

persistent Cnt
if(isempty(Cnt))
    Cnt = 0;
end

if (IsNear(Cnt, 0))
    MAPValid = boolean(true);  % init_MAPflag = 0 자동출력 방지
    Cnt = Cnt + 1;
else
    MAPValid = In_MAPValid;
end

function tf=IsNear(a,b,tol)
%ISNEAR True Where Nearly Equal.
% ISNEAR(A,B) returns a logical array the same size as A and B that is True
% where A and B are almost equal to each other and False where they are not.
% A and B must be the same size or one can be a scalar.
% ISNEAR(A,B,TOL) uses the tolerance TOL to determine nearness. In this
% case, TOL can be a scalar or an array the same size as A and B.
%
% When TOL is not provided, TOL = SQRT(eps).
%
% Use this function instead of A==B when A and B contain noninteger values.
% D.C. Hanselman, University of Maine, Orono, ME 04469
% Mastering MATLAB 7
% 2005-03-09
%--------------------------------------------------------------------------
if nargin==2
%    tol=sqrt(eps);       % original version
	tol=sqrt(eps(max(abs(a),abs(b))));     %  my version. sqrt seems like 'overdamping'
end
% when in need of optimization, drop the error checks
if ~isnumeric(a) || isempty(a) || ~isnumeric(b) || isempty(b) ||...
   ~isnumeric(tol) || isempty(tol)
   error('Inputs Must be Numeric.')
end
if any(size(a)~=size(b)) && numel(a)>1 && numel(b)>1
   error('A and B Must be the Same Size or Either can be a Scalar.')
end
% main line
tf=abs((a-b))<=abs(tol);

== matlab function TRN_V3_2/TRN/ModeManagementCSU/AcquisitionCSU/AcquisitionCSU/SetProfile ==
  data: batchProfile input; batchProfile output; profileCnt input; profileCnt output; gridSize input; gridSize output; profileLimit input
function [batchProfile, profileCnt, gridSize] = SetProfile(batchProfile, profileCnt, gridSize, profileLimit)

if(profileCnt >= profileLimit)

    profileCnt = uint32(profileLimit-1);

    for i = 0:profileCnt-1

        for j = 1 : (3 + (gridSize + gridSize + 1) * (gridSize + gridSize + 1))
            batchProfile(i * (3 + (gridSize + gridSize + 1) * (gridSize + gridSize + 1)) + j) = batchProfile((i+1) * (3 + (gridSize + gridSize + 1) * (gridSize + gridSize + 1)) + j);
        end
    end

end

end

== matlab function TRN_V3_2/TRN/TRN_visualization/Subsystem/MATLAB Function1 ==
  data: y input; x input; a output
function a = fcn(y,x)

a = sqrt(x^2+y^2);

== matlab function TRN_V3_2/TRN/TRN_visualization/Subsystem/Terrain_Level_big4 ==
  data: Lat input; Lon input; R output
function R = Terrain_level_big1(Lat, Lon)

    R = Terrain_level(Lat, Lon);

end

== matlab function TRN_V3_2/TRN/TRN_visualization/Subsystem1/MATLAB Function ==
  data: Err_Lat_INS output; Err_Lon_INS output; Err_Alt_INS output; lat_Ref input; lon_Ref input; alt_Ref input; lat_INS input; lon_INS input; alt_INS input; Lat_INS output; Lon_INS output; Alt_INS output; Lat_Ref output; Lon_Ref output; Alt_Ref output
function [Err_Lat_INS, Err_Lon_INS, Err_Alt_INS, Lat_INS, Lon_INS, Alt_INS, Lat_Ref, Lon_Ref, Alt_Ref] = fcn(lat_Ref, lon_Ref, alt_Ref, lat_INS, lon_INS, alt_INS)

%% parameters
lat2m = 110961.7060516;
lon2m = 89476.51124;

%% 초기값 setting
% init_lat = 35.1;
% init_lon = 128.5;
% init_alt = 1000;

Lat_INS = lat_INS;               % INS Latitude
Lon_INS = lon_INS;               % INS Longitude
% Alt_INS = uint16(alt_INS);               % INS Altitude
Alt_INS = alt_INS;               % INS Altitude

Lat_Ref = lat_Ref;             % Ref Latitude
Lon_Ref = lon_Ref;             % Ref Longitude
% Alt_Ref = uint16(alt_Ref);             % Ref Altitude
Alt_Ref = alt_Ref;             % Ref Altitude

Err_Lat_INS = (Lat_Ref-Lat_INS)*lat2m;
Err_Lon_INS = (Lon_Ref-Lon_INS)*lon2m;
Err_Alt_INS = (Alt_Ref-Alt_INS);

end

== matlab function TRN_V3_2/TRN/TRN_visualization/Subsystem3/MATLAB Function1 ==
  data: y input; x input; a output
function a = fcn(y,x)

a = sqrt(x^2+y^2);

== matlab function TRN_V3_2/TRN/TRN_visualization/Subsystem3/Terrain_Level_big4 ==
  data: Lat input; Lon input; R output
function R = Terrain_level_big1(Lat, Lon)

    R = Terrain_level(Lat, Lon);

end

== matlab function TRN_V3_2/TRN/TRN_visualization/Subsystem4/MATLAB Function ==
  data: Err_Lat_INS output; Err_Lon_INS output; Err_Alt_INS output; lat_Ref input; lon_Ref input; alt_Ref input; lat_INS input; lon_INS input; alt_INS input; Lat_INS output; Lon_INS output; Alt_INS output; Lat_Ref output; Lon_Ref output; Alt_Ref output
function [Err_Lat_INS, Err_Lon_INS, Err_Alt_INS, Lat_INS, Lon_INS, Alt_INS, Lat_Ref, Lon_Ref, Alt_Ref] = fcn(lat_Ref, lon_Ref, alt_Ref, lat_INS, lon_INS, alt_INS)

%% parameters
lat2m = 110961.7060516;
lon2m = 89476.51124;

%% 초기값 setting
% init_lat = 35.1;
% init_lon = 128.5;
% init_alt = 1000;

Lat_INS = lat_INS;               % INS Latitude
Lon_INS = lon_INS;               % INS Longitude
% Alt_INS = uint16(alt_INS);               % INS Altitude
Alt_INS = alt_INS;               % INS Altitude

Lat_Ref = lat_Ref;             % Ref Latitude
Lon_Ref = lon_Ref;             % Ref Longitude
% Alt_Ref = uint16(alt_Ref);             % Ref Altitude
Alt_Ref = alt_Ref;             % Ref Altitude

Err_Lat_INS = (Lat_Ref-Lat_INS)*lat2m;
Err_Lon_INS = (Lon_Ref-Lon_INS)*lon2m;
Err_Alt_INS = (Alt_Ref-Alt_INS);

end

== matlab function TRN_V3_2/TRN/TRNvalidCheck ==
  data: INS_Mech_flag input; TRN_valid output; Latitude_INS input
function TRN_valid = TRNvalidCheck(INS_Mech_flag, Latitude_INS)

    if( abs(Latitude_INS) > 80.0)
        Latitude_INS_flag = 0;
    else
        Latitude_INS_flag = 1;
    end

    if( (INS_Mech_flag < 1) || (Latitude_INS_flag < 1))
        TRN_valid = boolean(false);
    else
        TRN_valid = boolean(true);
    end

end

== matlab function TRN_V3_2/TRN/Terrain_Func/CheckOffTerrainMap ==
  data: hDEM input; AircraftOffTerrainMap output
function AircraftOffTerrainMap = CheckOffTerrainMap(hDEM)

if (IsNear(hDEM, -1.0))
    AircraftOffTerrainMap = true;
else
    AircraftOffTerrainMap = false;
end

end

function tf=IsNear(a,b,tol)
%ISNEAR True Where Nearly Equal.
% ISNEAR(A,B) returns a logical array the same size as A and B that is True
% where A and B are almost equal to each other and False where they are not.
% A and B must be the same size or one can be a scalar.
% ISNEAR(A,B,TOL) uses the tolerance TOL to determine nearness. In this
% case, TOL can be a scalar or an array the same size as A and B.
%
% When TOL is not provided, TOL = SQRT(eps).
%
% Use this function instead of A==B when A and B contain noninteger values.
% D.C. Hanselman, University of Maine, Orono, ME 04469
% Mastering MATLAB 7
% 2005-03-09
%--------------------------------------------------------------------------
if nargin==2
%    tol=sqrt(eps);       % original version
	tol=sqrt(eps(max(abs(a),abs(b))));     %  my version. sqrt seems like 'overdamping'
end
% when in need of optimization, drop the error checks
if ~isnumeric(a) || isempty(a) || ~isnumeric(b) || isempty(b) ||...
   ~isnumeric(tol) || isempty(tol)
   error('Inputs Must be Numeric.')
end
if any(size(a)~=size(b)) && numel(a)>1 && numel(b)>1
   error('A and B Must be the Same Size or Either can be a Scalar.')
end
% main line
tf=abs((a-b))<=abs(tol);
end

== matlab function TRN_V3_2/TRN/Terrain_Func/FTGMapCaching ==
  data: resultDTED output; resultDVOF output; lat input; lon input; hDEM output
function [resultDTED, resultDVOF, hDEM] = FTGMapCaching(lat, lon)

resultDTED = uint32(1);
resultDVOF = int32(1);
hDEM = double(0.0);                                 %%20220419

resultDTED = coder.ceval('UpdateCache', lat, lon);
hDEM = coder.ceval('MAPGetTerrainHeight', lat, lon);       %%20220419

== matlab function TRN_V3_2/TRN/Terrain_Func/Terrain_Level_big ==
  data: Lat input; Lon input; R output
function R = Terrain_level_big(Lat, Lon)

    R = Terrain_level(Lat, Lon);

end

== matlab function TRN_V3_2/TRN/Terrain_Func/updateFlag ==
  data: AircraftOffTerrainMap input; roughness input; UpdateFlag output
function UpdateFlag = updateFlag(AircraftOffTerrainMap, roughness)

persistent NotupdateCnt
if(isempty(NotupdateCnt))
    NotupdateCnt = 0;
end

if roughness < 1
    NotupdateCnt = NotupdateCnt + 0.04;
else
    NotupdateCnt = 0;
end

if AircraftOffTerrainMap == true || NotupdateCnt > 10 * 60   % 10 min
    UpdateFlag = 0;
else
    UpdateFlag = 1;
end

== matlab function TRN_V3_2/TRN/ModeManagementCSU/TrackingCSU/TrackingCSU_20230430/TrackingCSU_ConvertInput1/MATLAB Function1 ==
  data: gV output; x input; flag output; y input
function [gV, flag] = Groundspeed(x,y)

limSpeed_low  = 100*0.514444;  % unit : m/s
limSpeed_high = 700*0.514444;  % unit : m/s

gV = sqrt(x^2+y^2);

if gV > limSpeed_low && gV < limSpeed_high
    flag = boolean(true);
else
    flag = boolean(false);
end

== matlab function TRN_V3_2/TRN/GPSmode_Uncertainty_init/Uncertainty_init ==
  data: hUncertainty output; vUncertainty output
function [hUncertainty,vUncertainty] = Uncertainty_init

R0      = 6378000;

attBias = [0 0 0];
velBias = [0 0 0];
posBias = [10 10 13.3] .* [1/R0 1/R0 1];
gyroBias = [0.4848e-6 0.4848e-6 0.4848e-6];
accBias = [2.9430e-4 2.9430e-4 2.9430e-4];

Pmat = diag([attBias velBias posBias gyroBias accBias].^2);

hUncertainty = sqrt(abs(Pmat(7,7) + Pmat(8,8))) * 6378000;
vUncertainty = sqrt(abs(Pmat(9,9)));
